simulink model "mslbus_05"  (Simulink 6.3)
settings: Solver=FixedStepDiscrete  StartTime=0.0  StopTime=10.0  RelTol=1e-3
CloseFcn:
  | rtwprivate ssgencode ModelCloseRequest prob1
settings Model: Creator=stoeppe  LastModifiedBy=mshakeri  ExtModeAutoUpdateStatusClock=off  StrictBusMsg=ErrorLevel1
settings DataIOCC: SaveFormat=StructureWithTime  SignalLoggingName=sigsOut
settings OptimizationCC: InlineParams=on  OptimizeModelRefInitCode=on  LifeSpan=1
settings DebuggingCC: SigSpecEnsureSampleTime=on  SignalResolutionControl=UseLocalSettings  SolverPrmCheckMsg=none
settings HardwareCC: TargetUnknown=on
settings RTWCC: SystemTargetFile=ert.tlc  GenCodeOnly=on  TemplateMakefile=ert_default_tmf  GenerateReport=on  ProcessScript=ert_make_rtw_hook  IncludeHyperlinkInReport=on  LaunchReport=on
settings CodeAppCC: IgnoreCustomStorageClasses=off
settings ERTTargetCC: TargetFcnLib=ansi_tfl_tmw.mat  GenFloatMathFcnCalls=ANSI_C  GenerateSampleERTMain=on  InlinedParameterPlacement=NonHierarchical  ERTCustomFileTemplate=example_file_process.tlc  InitialValueSource=Model

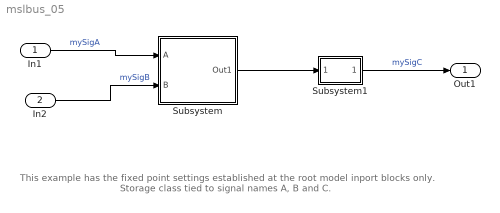
== system mslbus_05 ==
  note: This example has the fixed point settings
      | established at the root model inport blocks only.
      | Storage class tied to signal names A, B and C.
  In1 : Inport  Port=1  DataType=Specify via dialog  OutScaling=0.34555643  LatchInput=off  HoldInput=off
  In2 : Inport  Port=2  DataType=Specify via dialog  OutScaling=2^7  LatchInput=off  HoldInput=off
  Subsystem : Subsystem  TreatAsAtomicUnit=on
      settings: RTWSystemCode=Function  RTWFcnNameOpts=Use subsystem name
  Subsystem1 : Subsystem
  Out1 : Outport
  wires:
  In1/1 -> Subsystem/1(A)  "mySigA"
  In2/1 -> Subsystem/2(B)  "mySigB"
  Subsystem/1(Out1) -> Subsystem1/1(In1)
  Subsystem1/1(Out1) -> Out1/1  "mySigC"

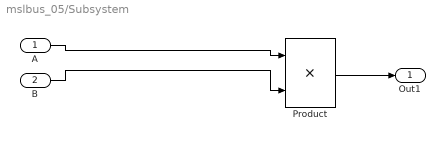
== system mslbus_05/Subsystem ==
  A : Inport  Port=1  LatchInput=off  HoldInput=off
  B : Inport  Port=2  LatchInput=off  HoldInput=off
  Product : Product  SaturateOnIntegerOverflow=on
  Out1 : Outport
  wires:
  B/1 -> Product/2
  A/1 -> Product/1
  Product/1 -> Out1/1

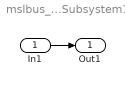
== system mslbus_05/Subsystem1 ==
  In1 : Inport  Port=1  LatchInput=off  HoldInput=off
  Out1 : Outport
  wires:
  In1/1 -> Out1/1
